simulink model "FSK"  (R2015b)
settings: Solver=VariableStepAuto  StartTime=0.0  StopTime=10.0  RelTol=1e-3
libraries: dspquant2 x1
settings Model: Creator=Administrator  LastModifiedBy=xiao'xin

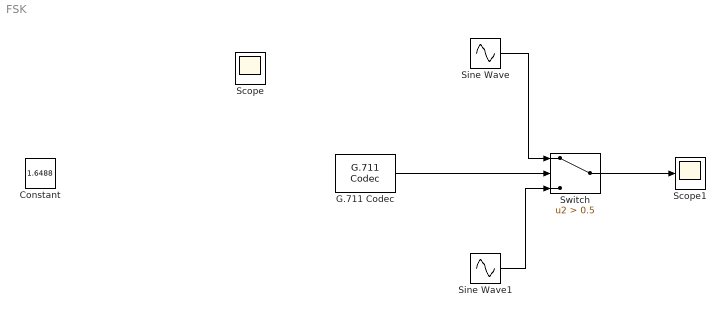
== system FSK ==
  Constant : Constant  Value=1.6488
  G.711 Codec : dspquant2/G.711 Codec  mode=Encode PCM to A-law  errmode=Warning
  Scope : Scope
  Scope1 : Scope
  Sine Wave : Sin  SampleTime=0
  Sine Wave1 : Sin  SampleTime=0
  Switch : Switch  Criteria=u2 > Threshold  Threshold=0.5
  wires:
  G.711 Codec/1 -> Switch/2
  Sine Wave/1 -> Switch/1
  Sine Wave1/1 -> Switch/3
  Switch/1 -> Scope1/1
